simulink model "step4_1_compare_lin_non_lin1"  (R2021b)
settings: Solver=VariableStepAuto  StartTime=0.0  StopTime=10.0  RelTol=1e-3
values from neighbouring files (symbols this model uses):
  A = double(A)    [Linearize.m]    (also in linearize_compare.m; step4_linearized_system.mat = [0 1.79155728996 0 -111.114105003 0 1 -687.855245355 0 1440.)
  B = double(B)    [Linearize.m]    (also in linearize_compare.m; step4_linearized_system.mat = [0 0 0 0 2553.84140127])
  b1 = params(10)    [Linearize.m]    (also in linearize_compare.m)
  b2 = params(11)    [Linearize.m]    (also in linearize_compare.m)
  C = [1  0  0  0  0; 0  0  1  0  0]    [Jacobian.mat]    (also in Linearize.m = double(C); linearize_compare.m = [1 0 0 0 0; step4_linearized_system.mat)
  c1 = params(6)    [Linearize.m]    (also in linearize_compare.m)
  c2 = params(7)    [Linearize.m]    (also in linearize_compare.m)
  D = [0 0]    [Jacobian.mat]    (also in Linearize.m = double(D); linearize_compare.m = zeros(2,1); step4_linearized_system.mat)
  g1 = (m1 * c1 + m2 * l1) * g    [Linearize.m]    (also in linearize_compare.m)
  g2 = m2 * c2 * g    [Linearize.m]    (also in linearize_compare.m)
  I1 = params(8)    [Linearize.m]    (also in linearize_compare.m)
  I2 = params(9)    [Linearize.m]    (also in linearize_compare.m)
  km = params(12)    [Linearize.m]    (also in linearize_compare.m)
  l1 = 0.1    [Linearize.m]    (also in linearize_compare.m = params(2))
  l2 = 0.1    [Linearize.m]    (also in linearize_compare.m = params(3))
  m1 = 0.125    [Linearize.m]    (also in linearize_compare.m = params(4))
  m2 = 0.05    [Linearize.m]    (also in linearize_compare.m = params(5))
  P1 = m1 * c1 * c1 + m2 * l1 * l1 + I1    [Linearize.m]    (also in linearize_compare.m)
  P2 = m2 * c2 * c2 + I2    [Linearize.m]    (also in linearize_compare.m)
  P3 = m2 * l1 * c2    [Linearize.m]    (also in linearize_compare.m)
  params = [0 0 0 0 0 params]    [Linearize.m]    (also in params.mat = [9.81 0.1 0.1 0.125 0.046955 -0.032 0.04609 0.0088 9.8e-05 6; sss.m = [9.81, 0.1, 0.1, 0.125, 0.046955, -0.032, 0.04609, 0.008800,; step4_linearized_system.mat = [9.81 0.1 0.1 0.125 0.046955 -0.032 0.04609 0.0088 9.8e-05 6)
  tau_e = params(13)    [Linearize.m]    (also in linearize_compare.m)
  theta_1_0 = pi    (= 3.14159265359)    [Linearize.m]    (also in linearize_compare.m)
  theta_2_0 = 0    [Linearize.m]    (also in linearize_compare.m)
  x_op = [theta_1_0; 0; theta_2_0; 0; 0]    [linearize_compare.m]    (also in step4_linearized_system.mat = [3.14159265359 0 0 0 0])
settings Model: LastModifiedBy=amavanmierlo
settings OptimizationCC: BlockReduction=off  BooleanDataType=off
settings DebuggingCC: SaveWithParameterizedLinksMsg=none  UnderspecifiedInitializationDetection=Classic  MergeDetectMultiDrivingBlocksExec=none  SignalResolutionControl=TryResolveAllWithWarning
settings HardwareCC: TargetUnknown=on
settings ModelReferenceCC: PropagateSignalLabelsOutOfModel=off

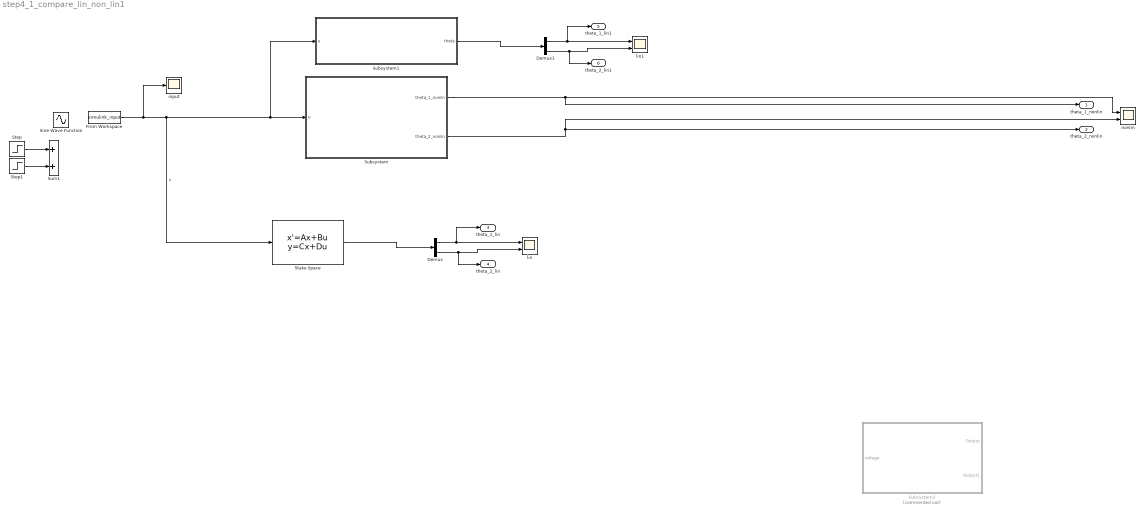
== system step4_1_compare_lin_non_lin1 ==
  Demux : Demux  Outputs=2
  Demux1 : Demux  Outputs=2
  From Workspace : FromWorkspace  SampleTime=-1
  Sine Wave Function : Sin  Amplitude=0.05  Frequency=2*pi*2  SampleTime=0.001
  State-Space : StateSpace  A=A  B=B  C=C  D=D  InitialCondition=x_op-x_op
  Step : Step  Time=0
  Step1 : Step  Time=0.05  After=-1
  Subsystem : Subsystem
  Subsystem1 : Subsystem
  Subsystem2 : Subsystem  Commented=on
  Sum1 : Sum
  input : Scope
  lin : Scope  NumInputPorts=2
  lin1 : Scope  NumInputPorts=2
  nonlin : Scope  NumInputPorts=2
  theta_1_nonlin : Outport
  theta_2_nonlin : Outport  Port=2
  theta_1_lin : Outport  Port=3
  theta_2_lin : Outport  Port=4
  theta_1_lin1 : Outport  Port=5
  theta_2_lin1 : Outport  Port=6
  wires:
  Demux/1 -> theta_1_lin/1, lin/1
  Demux/2 -> lin/2, theta_2_lin/1
  State-Space/1 -> Demux/1
  Step1/1 -> Sum1/2
  Step/1 -> Sum1/1
  From Workspace/1 -> State-Space/1, Subsystem/1(u), Subsystem1/1(u), input/1  "u"
  Subsystem/1(theta_1_nonlin) -> theta_1_nonlin/1, nonlin/1
  Subsystem/2(theta_2_nonlin) -> nonlin/2, theta_2_nonlin/1
  Demux1/1 -> theta_1_lin1/1, lin1/1
  Demux1/2 -> lin1/2, theta_2_lin1/1
  Subsystem1/1(theta) -> Demux1/1

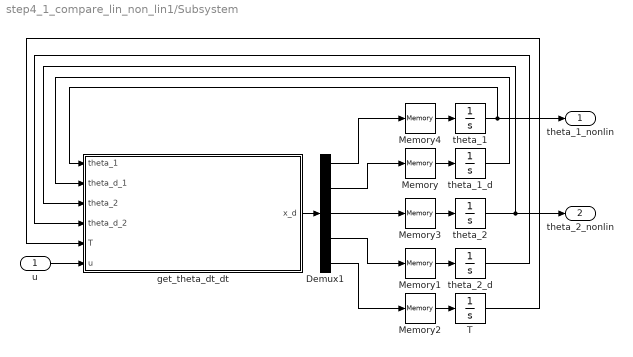
== system step4_1_compare_lin_non_lin1/Subsystem ==
  u : Inport
  Demux1 : Demux  Outputs=5
  Memory{,1..4} (5 alike) : Memory
  T : Integrator
  get_theta_dt_dt : MATLAB Function  TreatAsAtomicUnit=on
  theta_1 : Integrator  InitialCondition=theta_1_0
  theta_1_d : Integrator
  theta_2 : Integrator  InitialCondition=theta_2_0
  theta_2_d : Integrator
  theta_1_nonlin : Outport
  theta_2_nonlin : Outport  Port=2
  wires:
  Demux1/2 -> Memory/1
  theta_1/1 -> theta_1_nonlin/1, get_theta_dt_dt/1(theta_1)
  u/1 -> get_theta_dt_dt/6(u)
  get_theta_dt_dt/1(x_d) -> Demux1/1
  Demux1/4 -> Memory1/1
  theta_1_d/1 -> get_theta_dt_dt/2(theta_d_1)
  theta_2/1 -> theta_2_nonlin/1, get_theta_dt_dt/3(theta_2)
  theta_2_d/1 -> get_theta_dt_dt/4(theta_d_2)
  T/1 -> get_theta_dt_dt/5(T)
  Memory/1 -> theta_1_d/1
  Memory1/1 -> theta_2_d/1
  Demux1/5 -> Memory2/1
  Memory2/1 -> T/1
  Memory3/1 -> theta_2/1
  Demux1/3 -> Memory3/1
  Memory4/1 -> theta_1/1
  Demux1/1 -> Memory4/1

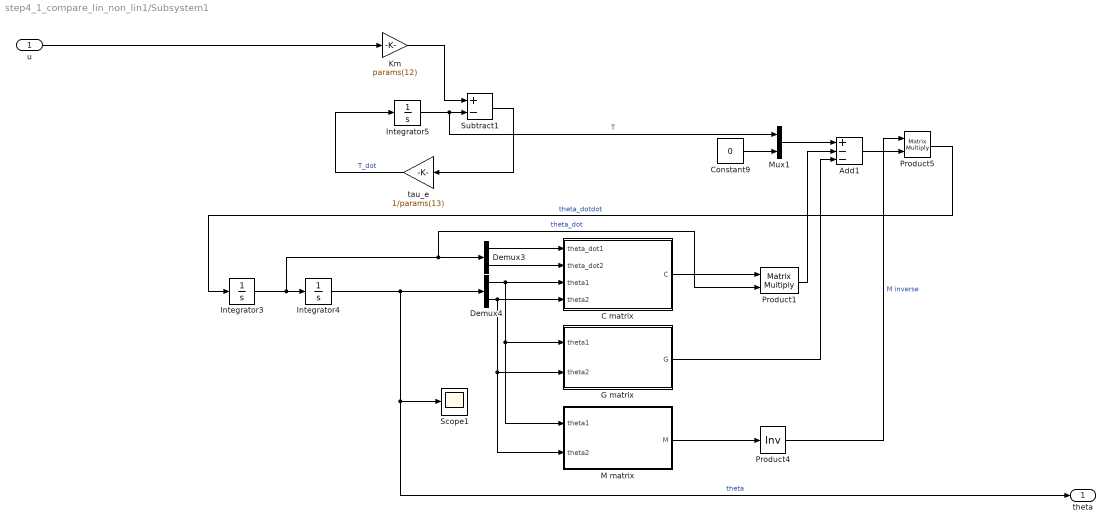
== system step4_1_compare_lin_non_lin1/Subsystem1 ==
  u : Inport
  Add1 : Sum  Inputs=+--
  C matrix : MATLAB Function  TreatAsAtomicUnit=on
  Constant9 : Constant  Value=0
  Demux3 : Demux  Outputs=2
  Demux4 : Demux  Outputs=2
  G matrix : MATLAB Function  TreatAsAtomicUnit=on
  Integrator3 : Integrator
  Integrator4 : Integrator  InitialCondition=[theta_1_0, theta_2_0]
  Integrator5 : Integrator
  Km : Gain  Gain=params(12)
  M matrix : MATLAB Function  TreatAsAtomicUnit=on
  Mux1 : Mux  Inputs=2
  Product1 : Product  Inputs=**  Multiplication=Matrix(*)
  Product4 : Product  Inputs=/  Multiplication=Matrix(*)
  Product5 : Product  Inputs=**  Multiplication=Matrix(*)
  Scope1 : Scope
  Subtract1 : Sum  Inputs=+-
  tau_e : Gain  Gain=1/params(13)
  theta : Outport
  wires:
  Demux4/1 -> M matrix/1(theta1), G matrix/1(theta1), C matrix/3(theta1)
  tau_e/1 -> Integrator5/1  "T_dot"
  Constant9/1 -> Mux1/2
  Demux3/1 -> C matrix/1(theta_dot1)
  Add1/1 -> Product5/2
  Subtract1/1 -> tau_e/1
  G matrix/1(G) -> Add1/3
  Integrator3/1 -> Product1/2, Demux3/1, Integrator4/1  "theta_dot"
  C matrix/1(C) -> Product1/1
  Mux1/1 -> Add1/1
  Integrator5/1 -> Mux1/1, Subtract1/2  "T"
  u/1 -> Km/1
  Product5/1 -> Integrator3/1  "theta_dotdot"
  Demux3/2 -> C matrix/2(theta_dot2)
  Integrator4/1 -> Demux4/1, theta/1, Scope1/1  "theta"
  M matrix/1(M) -> Product4/1
  Demux4/2 -> M matrix/2(theta2), G matrix/2(theta2), C matrix/4(theta2)
  Product4/1 -> Product5/1  "M inverse"
  Product1/1 -> Add1/2
  Km/1 -> Subtract1/1

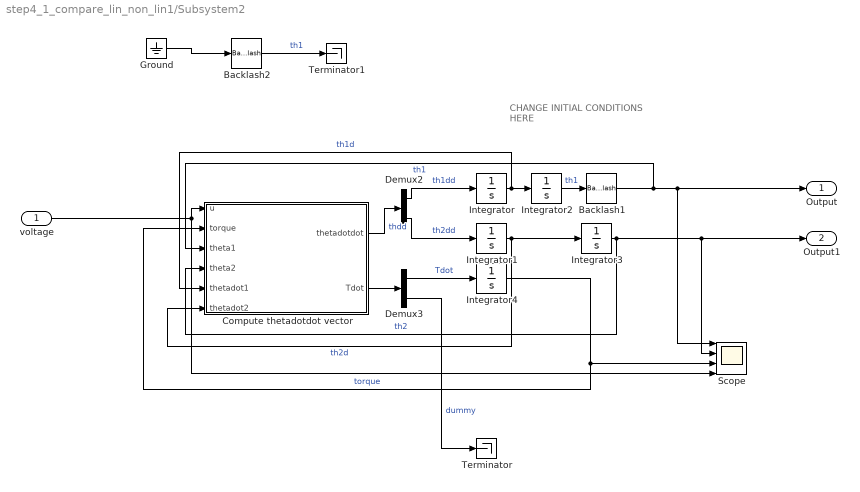
== system step4_1_compare_lin_non_lin1/Subsystem2 ==
  note: CHANGE INITIAL CONDITIONS HERE
  voltage : Inport
  Backlash1 : Backlash  BacklashWidth=0.0087
  Backlash2 : Backlash  BacklashWidth=0.0087
  Compute thetadotdot vector : MATLAB Function  TreatAsAtomicUnit=on
  Demux2 : Demux  Outputs=2
  Demux3 : Demux  Outputs=2
  Ground : Ground
  Integrator : Integrator
  Integrator1 : Integrator
  Integrator2 : Integrator  InitialCondition=theta_1_0
  Integrator3 : Integrator  InitialCondition=theta_2_0
  Integrator4 : Integrator
  Scope : Scope  NumInputPorts=4
  Terminator : Terminator
  Terminator1 : Terminator
  Output : Outport
  Output1 : Outport  Port=2
  wires:
  Demux2/1 -> Integrator/1  "th1dd"
  voltage/1 -> Scope/4, Compute thetadotdot vector/1(u)
  Backlash1/1 -> Compute thetadotdot vector/3(theta1), Output/1, Scope/1  "th1"
  Demux3/2 -> Terminator/1  "dummy"
  Demux2/2 -> Integrator1/1  "th2dd"
  Integrator/1 -> Compute thetadotdot vector/5(thetadot1), Integrator2/1  "th1d"
  Integrator1/1 -> Compute thetadotdot vector/6(thetadot2), Integrator3/1  "th2d"
  Demux3/1 -> Integrator4/1  "Tdot"
  Integrator2/1 -> Backlash1/1  "th1"
  Integrator3/1 -> Output1/1, Scope/2, Compute thetadotdot vector/4(theta2)  "th2"
  Compute thetadotdot vector/1(thetadotdot) -> Demux2/1  "thdd"
  Ground/1 -> Backlash2/1
  Backlash2/1 -> Terminator1/1  "th1"
  Compute thetadotdot vector/2(Tdot) -> Demux3/1
  Integrator4/1 -> Scope/3, Compute thetadotdot vector/2(torque)  "torque"

== matlab function step4_1_compare_lin_non_lin1/Subsystem2/Compute thetadotdot vector ==
  data: u input; torque input; thetadotdot output; theta1 input; theta2 input; thetadot1 input; thetadot2 input; l1 parameter; l2 parameter; m1 parameter; m2 parameter; c1 parameter; c2 parameter; I1 parameter; I2 parameter; b1 parameter; b2 parameter; km parameter; Tdot output; tau_e parameter
function [thetadotdot, Tdot]  = get_thetadotdot(u, torque, theta1, theta2, thetadot1, thetadot2, l1, l2, m1, m2, c1, c2, I1, I2, b1, b2, km, tau_e)
%% Parameters (SI Units)
g = 9.81;
%% Variables of the model
th1 = theta1;
th2 = theta2;
th1d = thetadot1;
th2d = thetadot2;
thd_vec = [th1d ; th2d];
thetadotdot = [0 ; 0];
T_vec = [torque ; 0];

%% Matrices of physical model
P1 = m1 * c1 * c1 + m2 * l1 * l1 + I1;
P2 = m2 * c2 * c2 + I2;
P3 = m2 * l1 * c2;
g1 = (m1 * c1 + m2 * l1) * g;
g2 = m2 * c2 * g;

M = [[P1 + P2 + 2*P3*cos(th2), P2 + P3 * cos(th2)]; [P2 + P3 * cos(th2) P2]];
C = [[b1 - P3 * th2d * sin(th2), -P3 * (th1d + th2d)*sin(th2)]; [P3 * th1d * sin(th2), b2]];
G = [- g1 * sin(th1) - g2 * sin(th1 + th2); - g2 * sin(th1 + th2)];

%% Compute output angular acceleration
M_inv = inv(M);
Tdot = (km*u - T_vec)/tau_e;
thetadotdot = M_inv*T_vec - M_inv*C*thd_vec - M_inv*G;

== matlab function step4_1_compare_lin_non_lin1/Subsystem1/C matrix ==
  data: theta_dot1 input; theta_dot2 input; theta1 input; theta2 input; C output; params parameter; P3 parameter
function C = C(theta_dot1, theta_dot2, theta1, theta2, params, P3)
c00 = params(10) - P3 * theta_dot2 * sin(theta2);
c01 = -P3 * (theta_dot1 + theta_dot2) * sin(theta2);
c10 = P3 * theta_dot1 * sin(theta2);
c11 = params(11);

C = [c00 c01;
     c10 c11];

== matlab function step4_1_compare_lin_non_lin1/Subsystem1/G matrix ==
  data: theta1 input; theta2 input; G output; g1 parameter; g2 parameter
function G = G(theta1, theta2, g1, g2)
G00 = -g1 * sin(theta1) - g2 * sin(theta1 + theta2);
G01 = -g2 * sin(theta1 + theta2);

G = [G00 G01];

== matlab function step4_1_compare_lin_non_lin1/Subsystem1/M matrix ==
  data: theta1 input; theta2 input; M output; P1 parameter; P2 parameter; P3 parameter
function M = fcn(theta1, theta2, P1, P2, P3)
M00 = P1 + P2 + 2 * P3 * cos(theta2);
M01 = P2 + P3 * cos(theta2);
M10 = M01;
M11 = P2;

M = [M00 M01;
     M10 M11];

== matlab function step4_1_compare_lin_non_lin1/Subsystem/get_theta_dt_dt ==
  settings: updateMethod=DISCRETE  sampleTime=0.001
  data: x_d output size=5; theta_1 input size=1; theta_d_1 input size=1; theta_2 input; theta_d_2 input size=1; T input; u input size=1
function x_d = get_theta_dt_dt(theta_1, theta_d_1, theta_2, theta_d_2, T, u)

% params = [-0.04, 0.06, 0.074, 0.00002, 4.8, 0.00077, 50, 0.03];
params = [0 -0.032, 0.04609, 0.088800, 0.000099, 6.301237, 0.000027, 40.09531, 0.01537];

% varying variables
c_1 = params(2);
c_2 = params(3);
I_1 = params(4);
I_2 = params(5);
b_1 = params(6);
b_2 = params(7);
k_m = params(8);
tau_e = params(9);


fun =  @(I_1,I_2,T,b_1,b_2,c_1,c_2,k_m,tau_e,theta_1,theta_2,theta_d_1,theta_d_2,u)[theta_d_1;-theta_d_1.*(((b_1-c_2.*theta_d_2.*sin(theta_2).*4.6955e-3).*(I_2.*3.602879701896397e+16+c_2.^2.*1.691732164025453e+15).*9.223372036854776e+18)./(I_2.*1.560347513552018e+32-c_2.^2.*cos(theta_2).^2.*7.326611749883501e+30+I_1.*c_2.^2.*1.560347513552018e+34+I_2.*c_1.^2.*4.153837486827862e+34+c_2.^2.*7.326611749883501e+30+c_1.^2.*c_2.^2.*1.950434391940023e+33+I_1.*I_2.*3.32306998946229e+35)-(c_2.*theta_d_1.*sin(theta_2).*(I_2.*5.764607523034235e+17+c_2.*cos(theta_2).*2.706771462440725e+15+c_2.^2.*2.706771462440725e+16).*2.706771462440725e+15)./(I_2.*1.560347513552018e+32-c_2.^2.*cos(theta_2).^2.*7.326611749883501e+30+I_1.*c_2.^2.*1.560347513552018e+34+I_2.*c_1.^2.*4.153837486827862e+34+c_2.^2.*7.326611749883501e+30+c_1.^2.*c_2.^2.*1.950434391940023e+33+I_1.*I_2.*3.32306998946229e+35))+theta_d_2.*((b_2.*(I_2.*5.764607523034235e+17+c_2.*cos(theta_2).*2.706771462440725e+15+c_2.^2.*2.706771462440725e+16).*5.764607523034235e+17)./(I_2.*1.560347513552018e+32-c_2.^2.*cos(theta_2).^2.*7.326611749883501e+30+I_1.*c_2.^2.*1.560347513552018e+34+I_2.*c_1.^2.*4.153837486827862e+34+c_2.^2.*7.326611749883501e+30+c_1.^2.*c_2.^2.*1.950434391940023e+33+I_1.*I_2.*3.32306998946229e+35)+(c_2.*sin(theta_2).*(I_2.*3.602879701896397e+16+c_2.^2.*1.691732164025453e+15).*(theta_d_1+theta_d_2).*4.33083433990516e+16)./(I_2.*1.560347513552018e+32-c_2.^2.*cos(theta_2).^2.*7.326611749883501e+30+I_1.*c_2.^2.*1.560347513552018e+34+I_2.*c_1.^2.*4.153837486827862e+34+c_2.^2.*7.326611749883501e+30+c_1.^2.*c_2.^2.*1.950434391940023e+33+I_1.*I_2.*3.32306998946229e+35))+((sin(theta_1).*(c_1.*(9.81e+2./8.0e+2)+4.6062855e-2)+c_2.*sin(theta_1+theta_2).*4.6062855e-1).*(I_2.*3.602879701896397e+16+c_2.^2.*1.691732164025453e+15).*9.223372036854776e+18)./(I_2.*1.560347513552018e+32-c_2.^2.*cos(theta_2).^2.*7.326611749883501e+30+I_1.*c_2.^2.*1.560347513552018e+34+I_2.*c_1.^2.*4.153837486827862e+34+c_2.^2.*7.326611749883501e+30+c_1.^2.*c_2.^2.*1.950434391940023e+33+I_1.*I_2.*3.32306998946229e+35)+(T.*(I_2.*3.602879701896397e+16+c_2.^2.*1.691732164025453e+15).*9.223372036854776e+18)./(I_2.*1.560347513552018e+32-c_2.^2.*cos(theta_2).^2.*7.326611749883501e+30+I_1.*c_2.^2.*1.560347513552018e+34+I_2.*c_1.^2.*4.153837486827862e+34+c_2.^2.*7.326611749883501e+30+c_1.^2.*c_2.^2.*1.950434391940023e+33+I_1.*I_2.*3.32306998946229e+35)-(c_2.*sin(theta_1+theta_2).*(I_2.*5.764607523034235e+17+c_2.*cos(theta_2).*2.706771462440725e+15+c_2.^2.*2.706771462440725e+16).*2.655342804654351e+17)./(I_2.*1.560347513552018e+32-c_2.^2.*cos(theta_2).^2.*7.326611749883501e+30+I_1.*c_2.^2.*1.560347513552018e+34+I_2.*c_1.^2.*4.153837486827862e+34+c_2.^2.*7.326611749883501e+30+c_1.^2.*c_2.^2.*1.950434391940023e+33+I_1.*I_2.*3.32306998946229e+35);theta_d_2;-theta_d_2.*((b_2.*(I_1.*1.152921504606847e+18+I_2.*1.152921504606847e+18+c_2.*cos(theta_2).*1.08270858497629e+16+c_1.^2.*1.441151880758559e+17+c_2.^2.*5.41354292488145e+16+5.41354292488145e+14).*2.882303761517117e+17)./(I_2.*1.560347513552018e+32-c_2.^2.*cos(theta_2).^2.*7.326611749883501e+30+I_1.*c_2.^2.*1.560347513552018e+34+I_2.*c_1.^2.*4.153837486827862e+34+c_2.^2.*7.326611749883501e+30+c_1.^2.*c_2.^2.*1.950434391940023e+33+I_1.*I_2.*3.32306998946229e+35)+(c_2.*sin(theta_2).*(theta_d_1+theta_d_2).*(I_2.*5.764607523034235e+17+c_2.*cos(theta_2).*2.706771462440725e+15+c_2.^2.*2.706771462440725e+16).*2.706771462440725e+15)./(I_2.*1.560347513552018e+32-c_2.^2.*cos(theta_2).^2.*7.326611749883501e+30+I_1.*c_2.^2.*1.560347513552018e+34+I_2.*c_1.^2.*4.153837486827862e+34+c_2.^2.*7.326611749883501e+30+c_1.^2.*c_2.^2.*1.950434391940023e+33+I_1.*I_2.*3.32306998946229e+35))+theta_d_1.*(((b_1-c_2.*theta_d_2.*sin(theta_2).*4.6955e-3).*(I_2.*5.764607523034235e+17+c_2.*cos(theta_2).*2.706771462440725e+15+c_2.^2.*2.706771462440725e+16).*5.764607523034235e+17)./(I_2.*1.560347513552018e+32-c_2.^2.*cos(theta_2).^2.*7.326611749883501e+30+I_1.*c_2.^2.*1.560347513552018e+34+I_2.*c_1.^2.*4.153837486827862e+34+c_2.^2.*7.326611749883501e+30+c_1.^2.*c_2.^2.*1.950434391940023e+33+I_1.*I_2.*3.32306998946229e+35)-(c_2.*theta_d_1.*sin(theta_2).*(I_1.*1.152921504606847e+18+I_2.*1.152921504606847e+18+c_2.*cos(theta_2).*1.08270858497629e+16+c_1.^2.*1.441151880758559e+17+c_2.^2.*5.41354292488145e+16+5.41354292488145e+14).*1.353385731220362e+15)./(I_2.*1.560347513552018e+32-c_2.^2.*cos(theta_2).^2.*7.326611749883501e+30+I_1.*c_2.^2.*1.560347513552018e+34+I_2.*c_1.^2.*4.153837486827862e+34+c_2.^2.*7.326611749883501e+30+c_1.^2.*c_2.^2.*1.950434391940023e+33+I_1.*I_2.*3.32306998946229e+35))-((sin(theta_1).*(c_1.*(9.81e+2./8.0e+2)+4.6062855e-2)+c_2.*sin(theta_1+theta_2).*4.6062855e-1).*(I_2.*5.764607523034235e+17+c_2.*cos(theta_2).*2.706771462440725e+15+c_2.^2.*2.706771462440725e+16).*5.764607523034235e+17)./(I_2.*1.560347513552018e+32-c_2.^2.*cos(theta_2).^2.*7.326611749883501e+30+I_1.*c_2.^2.*1.560347513552018e+34+I_2.*c_1.^2.*4.153837486827862e+34+c_2.^2.*7.326611749883501e+30+c_1.^2.*c_2.^2.*1.950434391940023e+33+I_1.*I_2.*3.32306998946229e+35)-(T.*(I_2.*5.764607523034235e+17+c_2.*cos(theta_2).*2.706771462440725e+15+c_2.^2.*2.706771462440725e+16).*5.764607523034235e+17)./(I_2.*1.560347513552018e+32-c_2.^2.*cos(theta_2).^2.*7.326611749883501e+30+I_1.*c_2.^2.*1.560347513552018e+34+I_2.*c_1.^2.*4.153837486827862e+34+c_2.^2.*7.326611749883501e+30+c_1.^2.*c_2.^2.*1.950434391940023e+33+I_1.*I_2.*3.32306998946229e+35)+(c_2.*sin(theta_1+theta_2).*(I_1.*1.152921504606847e+18+I_2.*1.152921504606847e+18+c_2.*cos(theta_2).*1.08270858497629e+16+c_1.^2.*1.441151880758559e+17+c_2.^2.*5.41354292488145e+16+5.41354292488145e+14).*1.327671402327176e+17)./(I_2.*1.560347513552018e+32-c_2.^2.*cos(theta_2).^2.*7.326611749883501e+30+I_1.*c_2.^2.*1.560347513552018e+34+I_2.*c_1.^2.*4.153837486827862e+34+c_2.^2.*7.326611749883501e+30+c_1.^2.*c_2.^2.*1.950434391940023e+33+I_1.*I_2.*3.32306998946229e+35);-(T-k_m.*u)./tau_e];

x_d = fun(I_1,I_2,T,b_1,b_2,c_1,c_2,k_m,tau_e,theta_1,theta_2,theta_d_1,theta_d_2,u);
